simulink model "myPid"  (R2016b)
settings: Solver=VariableStepAuto  StartTime=0.0  StopTime=10.0  RelTol=1e-3
values from neighbouring files (symbols this model uses):
  tfPendDen = cell2mat(tfPend.Denominator)    [LCSproject.m]
  tfPendNum = cell2mat(tfPend.Numerator)    [LCSproject.m]
libraries: simulink x1
settings Model: Creator=Olivier  LastModifiedBy=Olivier

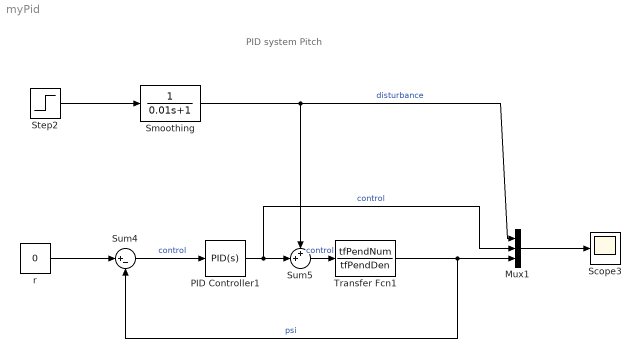
== system myPid ==
  note: PID system Pitch
  Mux1 : Mux  Inputs=3
  PID Controller1 : simulink/Continuous/PID Controller  Controller=PID  TimeDomain=Continuous-time  SampleTime=-1  IntegratorMethod=Forward Euler  FilterMethod=Forward Euler  Form=Parallel  UseFilter=on  ControllerParametersSource=internal  P=79.9541370836856  I=125.400260140081  D=8.23681666758394  N=3215.38634570315  InitialConditionSource=internal  InitialConditionForIntegrator=0  InitialConditionForFilter=0  ExternalReset=none  LimitOutput=off  UpperSaturationLimit=inf  LowerSaturationLimit=-inf  LinearizeAsGain=on  AntiWindupMode=none  Kb=1  TrackingMode=off  Kt=1  PParamMin=[]  PParamMax=[]  IParamMin=[]  IParamMax=[]  DParamMin=[]  DParamMax=[]  NParamMin=[]  NParamMax=[]  KbParamMin=[]  KbParamMax=[]  KtParamMin=[]  KtParamMax=[]  POutMin=[]  POutMax=[]  IOutMin=[]  IOutMax=[]  DOutMin=[]  DOutMax=[]  NOutMin=[]  NOutMax=[]  KbOutMin=[]  KbOutMax=[]  KtOutMin=[]  KtOutMax=[]  IntegratorOutMin=[]  IntegratorOutMax=[]  FilterOutMin=[]  FilterOutMax=[]  SumOutMin=[]  SumOutMax=[]  SumI1OutMin=[]  SumI1OutMax=[]  SumI2OutMin=[]  SumI2OutMax=[]  SumI3OutMin=[]  SumI3OutMax=[]  SumDOutMin=[]  SumDOutMax=[]  SaturationOutMin=[]  SaturationOutMax=[]  IntegratorContinuousStateAttributes=''  IntegratorStateMustResolveToSignalObject=off  IntegratorRTWStateStorageClass=Auto  FilterContinuousStateAttributes=''  FilterStateMustResolveToSignalObject=off  FilterRTWStateStorageClass=Auto  DifferentiatorICPrevScaledInput=0  DifferentiatorOutMin=[]  DifferentiatorOutMax=[]
  Scope3 : Scope
  "Smoothing " : TransferFcn  Denominator=[0.01 1]
  Step2 : Step  SampleTime=0
  Sum4 : Sum  Inputs=|+-
  Sum5 : Sum  Inputs=++|
  Transfer Fcn1 : TransferFcn  Numerator=tfPendNum  Denominator=tfPendDen
  r : Constant  Value=0
  wires:
  Sum4/1 -> PID Controller1/1  "control"
  Transfer Fcn1/1 -> Mux1/3, Sum4/2  "psi"
  Mux1/1 -> Scope3/1
  Step2/1 -> "Smoothing "/1
  PID Controller1/1 -> Mux1/2, Sum5/2  "control"
  Sum5/1 -> Transfer Fcn1/1  "control"
  "Smoothing "/1 -> Mux1/1, Sum5/1  "disturbance"
  r/1 -> Sum4/1
